simulink model "k1visbs_20170206"  (Simulink 8.5)
settings: Solver=ode45  StartTime=0.0  StopTime=10.0  RelTol=1e-3
libraries: cdsCDI64 x2, cdsCDO64 x2, cdsAdcx0 x1, TYPEB_MASTER x1, dac x1, cdsParameters x1
settings Model: Creator=keiko  LastModifiedBy=controls
settings DataIOCC: SignalLoggingSaveFormat=Dataset
settings OptimizationCC: ExpressionDepthLimit=128
settings DebuggingCC: UnderspecifiedInitializationDetection=Simplified  MergeDetectMultiDrivingBlocksExec=error  SolverPrmCheckMsg=warning  FcnCallInpInsideContextMsg=EnableAllAsError  StateNameClashWarn=none
settings GRTTargetCC: CombineOutputUpdateFcns=on  GRTInterface=off

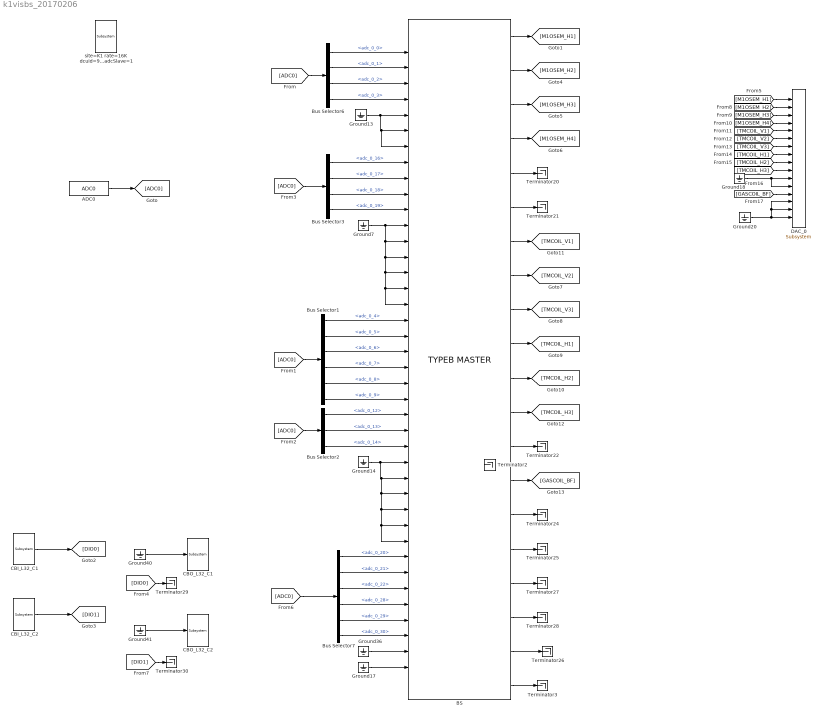
== system k1visbs_20170206 ==
  ADC0 : cdsAdcx0/ADC0  Tag=cdsAdc  Description=|
      | type-GSC_16AI64SSA
      | card_num=0
      settings: AttributesFormatString=%<Description>\n%<Tag>
  BS : TYPEB_MASTER/TYPEB MASTER  Description=TYPEB MASTER
      settings: AttributesFormatString=%<Description>
  Bus Selector1 : BusSelector  Description=ADC Selector  OutputSignals=adc_0_4,adc_0_5,adc_0_6,adc_0_7,adc_0_8,adc_0_9
      settings: AttributesFormatString=%<Description>
  Bus Selector2 : BusSelector  Description=ADC Selector  OutputSignals=adc_0_12,adc_0_13,adc_0_14
      settings: AttributesFormatString=%<Description>
  Bus Selector3 : BusSelector  Description=ADC Selector  OutputSignals=adc_0_16,adc_0_17,adc_0_18,adc_0_19
      settings: AttributesFormatString=%<Description>
  Bus Selector6 : BusSelector  Description=ADC Selector  OutputSignals=adc_0_0,adc_0_1,adc_0_2,adc_0_3
      settings: AttributesFormatString=%<Description>
  Bus Selector7 : BusSelector  Description=ADC Selector  OutputSignals=adc_0_20,adc_0_21,adc_0_22,adc_0_28,adc_0_29,adc_0_30
      settings: AttributesFormatString=%<Description>
  CBI_L32_C1 : cdsCDI64/Subsystem  Tag=cdsCDI64  Description=card_num=0
      settings: AttributesFormatString=%<Tag>\n%<Description>
  CBI_L32_C2 : cdsCDI64/Subsystem  Tag=cdsCDI64  Description=card_num=2
      settings: AttributesFormatString=%<Tag>\n%<Description>
  CBO_L32_C1 : cdsCDO64/Subsystem  Tag=cdsCDO64  Description=card_num=0
      settings: AttributesFormatString=%<Tag>\n%<Description>
  CBO_L32_C2 : cdsCDO64/Subsystem  Tag=cdsCDO64  Description=card_num=2
      settings: AttributesFormatString=%<Tag>\n%<Description>
  DAC_0 : dac/Subsystem  Description=|
      | type=GSC_16AO16,
      | card_num=0
      settings: AttributesFormatString=%<Description>
  Ground{7,13..14,17..18,20,36,40..41} (9 alike) : Ground
  Terminator{2..3,20..22,24..30} (12 alike) : Terminator
  site=K1 rate=16K dcuid=96 host=k1pr2 specific_cpu=4 adcSlave=1 : cdsParameters/Subsystem  Tag=cdsParameters  Description=|
      | Purpose:                                                                                                                                                                                                                                
      | Provide system parameters to the FE code generator to properly configure the generated EPICS names, rep rate of the FE controller, and the Data Acquisition node ID for proper storage of data from this FE controller.                 
      |                                                                                                                                                                                                                                         
      | Useage:                                                                                                                                                                                                                                 
      | The part NAME field is used to identify the FE parameters. It must be of the form:                                                                                                                                                      
      | site=                                                                                                                                                                                                                                   
      | rate=                                                                                                                                                                                                                                   
      | dcuid=                                                                                                                                                                                                                                  
      |                                                                                                                                                                                                                                         
      | Where:                                                                                                                                                                                                                                  
      | site= argument may be H1, H2, L1, M1, G1, either as a single argument or multiple, for example site=H1,H2. These are the only names allowed. These will become the first two characters of all EPICS and signal names (for example G1:).
      |                                                                                                                                                                                                                                         
      | rate= may be 2K, 16K, 32K, or 64K                                                                                                                                                                                                       
      |                                                                                                                                                                                                                                         
      | dcuid= is site specific ie it must be unique at each site.
      settings: AttributesFormatString=%<Tag>
  wires:
  ADC0/1 -> [ADC0]
  [ADC0] -> Bus Selector6/1
  [ADC0] -> Bus Selector1/1
  Bus Selector6/1 -> BS/1  "<adc_0_0>"
  Bus Selector6/2 -> BS/2  "<adc_0_1>"
  Bus Selector6/3 -> BS/3  "<adc_0_2>"
  Bus Selector6/4 -> BS/4  "<adc_0_3>"
  Bus Selector3/4 -> BS/11  "<adc_0_19>"
  Ground7/1 -> BS/12, BS/13, BS/14, BS/15, BS/17, BS/16
  Ground13/1 -> BS/5, BS/7, BS/6
  Bus Selector3/1 -> BS/8  "<adc_0_16>"
  Bus Selector3/3 -> BS/10  "<adc_0_18>"
  Bus Selector3/2 -> BS/9  "<adc_0_17>"
  Bus Selector1/1 -> BS/18  "<adc_0_4>"
  Bus Selector1/2 -> BS/19  "<adc_0_5>"
  Bus Selector1/3 -> BS/20  "<adc_0_6>"
  Bus Selector1/4 -> BS/21  "<adc_0_7>"
  Bus Selector1/5 -> BS/22  "<adc_0_8>"
  Bus Selector1/6 -> BS/23  "<adc_0_9>"
  Ground14/1 -> BS/27, BS/28, BS/29, BS/30, BS/32, BS/31
  [ADC0] -> Bus Selector2/1
  Bus Selector2/1 -> BS/24  "<adc_0_12>"
  [ADC0] -> Bus Selector3/1
  BS/5 -> Terminator20/1
  BS/6 -> Terminator21/1
  Ground17/1 -> BS/40
  Bus Selector2/2 -> BS/25  "<adc_0_13>"
  Bus Selector2/3 -> BS/26  "<adc_0_14>"
  BS/14 -> [GASCOIL_BF]
  BS/15 -> Terminator24/1
  BS/16 -> Terminator25/1
  BS/19 -> Terminator26/1
  BS/17 -> Terminator27/1
  BS/18 -> Terminator28/1
  [ADC0] -> Bus Selector7/1
  Ground36/1 -> BS/39
  Bus Selector7/1 -> BS/33  "<adc_0_20>"
  Bus Selector7/5 -> BS/37  "<adc_0_29>"
  Bus Selector7/6 -> BS/38  "<adc_0_30>"
  Bus Selector7/3 -> BS/35  "<adc_0_22>"
  Bus Selector7/2 -> BS/34  "<adc_0_21>"
  Bus Selector7/4 -> BS/36  "<adc_0_28>"
  CBI_L32_C1/1 -> [DIO0]
  CBI_L32_C2/1 -> [DIO1]
  Ground40/1 -> CBO_L32_C1/1
  Ground41/1 -> CBO_L32_C2/1
  [DIO0] -> Terminator29/1
  [DIO1] -> Terminator30/1
  BS/20 -> Terminator3/1
  Ground18/1 -> DAC_0/12, DAC_0/11
  Ground20/1 -> DAC_0/16, DAC_0/15, DAC_0/14
  BS/13 -> Terminator22/1
  BS/1 -> [M1OSEM_H1]
  BS/2 -> [M1OSEM_H2]
  BS/3 -> [M1OSEM_H3]
  BS/4 -> [M1OSEM_H4]
  [M1OSEM_H1] -> DAC_0/1
  [M1OSEM_H2] -> DAC_0/2
  [M1OSEM_H3] -> DAC_0/3
  [M1OSEM_H4] -> DAC_0/4
  BS/7 -> [TMCOIL_V1]
  BS/8 -> [TMCOIL_V2]
  BS/9 -> [TMCOIL_V3]
  BS/10 -> [TMCOIL_H1]
  BS/11 -> [TMCOIL_H2]
  BS/12 -> [TMCOIL_H3]
  [TMCOIL_V1] -> DAC_0/5
  [TMCOIL_V2] -> DAC_0/6
  [TMCOIL_V3] -> DAC_0/7
  [TMCOIL_H1] -> DAC_0/8
  [TMCOIL_H2] -> DAC_0/9
  [TMCOIL_H3] -> DAC_0/10
  [GASCOIL_BF] -> DAC_0/13
